simulink model "verify_Storage_Type_1_CONF_mdl"  (R2016b)
settings: Solver=ode45  StartTime=0  StopTime=24*3600  MaxStep=600  RelTol=1e-3  EnableMultiTasking=on
undefined symbols (not defined in the file or in its folder): path_carnot
libraries: carnot x7, simulink x2
settings Model: Creator=drhf  LastModifiedBy=drhf
settings DataIOCC: SaveFormat=Array  SignalLoggingSaveFormat=ModelDataLogs
settings OptimizationCC: ExpressionDepthLimit=2147483647  LifeSpan=inf
settings DebuggingCC: UnderspecifiedInitializationDetection=Classic  MergeDetectMultiDrivingBlocksExec=none  SolverPrmCheckMsg=warning  FcnCallInpInsideContextMsg=warning  StateNameClashWarn=warning  SFUnexpectedBacktrackingDiag=warning  SFNoUnconditionalDefaultTransitionDiag=warning  SFExecutionAtInitializationDiag=none
settings HardwareCC: ProdBitPerPointer=32  ProdBitPerSizeT=32  ProdBitPerPtrDiffT=32  ProdLargestAtomicFloat=None  ProdIntDivRoundTo=Undefined  ProdEndianess=Unspecified  ProdWordSize=32  ProdHWDeviceType=32-bit Generic
settings ModelReferenceCC: PropagateSignalLabelsOutOfModel=off
settings GRTTargetCC: TargetLangStandard=C89/C90 (ANSI)  GeneratePreprocessorConditionals=Disable all  CombineOutputUpdateFcns=off  GRTInterface=on
settings ConfigComp: CovMetricSettings=dw  CovHtmlReporting=on  CovSaveCumulativeToWorkspaceVar=on  CovSaveSingleToWorkspaceVar=on  CovExternalEMLEnable=off

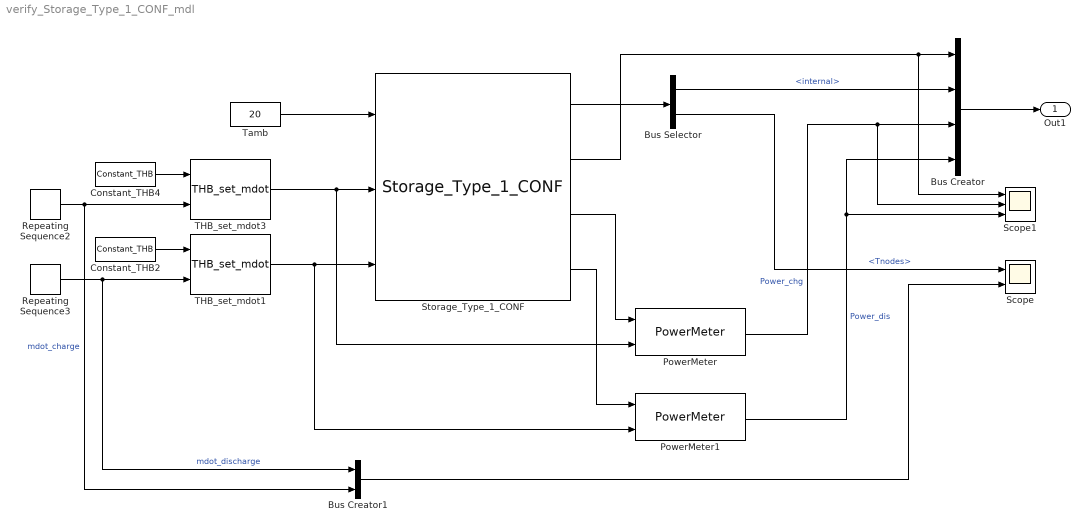
== system verify_Storage_Type_1_CONF_mdl ==
  Bus Creator : BusCreator  Inputs=4
  Bus Creator1 : BusCreator  Inputs=2
  Bus Selector : BusSelector  OutputSignals=energy.internal,Tnodes
  Constant_THB2 : carnot/Source/Simple/Constant_THB  t=10  mdot=100/3600  p=1e5  mID=Full Pressure Drop with Static Height  fluid=Water  mix=0  mix2=0  mix3=0  dia=0.02  hgt=0
  Constant_THB4 : carnot/Source/Simple/Constant_THB  t=55  mdot=0*100/3600  p=1e5  mID=Full Pressure Drop with Static Height  fluid=Water  mix=0  mix2=0  mix3=0  dia=0.02  hgt=0
  PowerMeter : carnot/Control/PowerMeter
  PowerMeter1 : carnot/Control/PowerMeter
  Repeating Sequence2 : simulink/Sources/Repeating Sequence  rep_seq_t=[ 0 3600 3600+eps(3600) 7200 7200+eps(7200) 10440 10440+eps(10440) 11160]  rep_seq_y=[ 0.12 0.12 0.15+0*eps(3600) 0.15 0.1+0*eps(7200) 0.1 0+0*eps(10440) 0]
  Repeating Sequence3 : simulink/Sources/Repeating Sequence  rep_seq_t=[ 0 3600 3600+eps(3600) 7200 7200+eps(7200) 10800]  rep_seq_y=[ 0.12 0.12 0.1+0*eps(3600) 0.1 0.15+0*eps(7200) 0.15]
  Scope : Scope  NumInputPorts=2
  Scope1 : Scope  NumInputPorts=3
  Storage_Type_1_CONF : carnot/Storage/Thermal/Storage_Type_1_CONF  t0=[10:5:55]  hgt=1.5279  stgtype=1  tini=[10 15 20 25 30 35 40 45 50 55]  mpts=[1 2 3 4 5 6 7 8 9 10]  PathName=fullfile(path_carnot('libsl'),'Storage','Thermal','Storage_Type_1_CONF','parameter_set')  FileName='StorageType1_300_L.mat'  userPath=off  userParam=off  uwall=1  ubot=1  utop=1  axcond=1  volume=0.3  dia=0.5  standing=standing cylinder  nodes=10  mpoints=10  Tsensor=0.5  pipe1inlet=1  pipe1outlet=0  pipe1dia=0.03  pipe2inlet=0  pipe2outlet=1  pipe2dia=0.03
  THB_set_mdot1 : carnot/Source/Simple/THB_set_mdot
  THB_set_mdot3 : carnot/Source/Simple/THB_set_mdot
  Tamb : Constant  Value=20
  Out1 : Outport
  wires:
  Bus Creator/1 -> Out1/1
  Tamb/1 -> Storage_Type_1_CONF/1
  THB_set_mdot1/1 -> Storage_Type_1_CONF/3, PowerMeter1/2
  Constant_THB2/1 -> THB_set_mdot1/1
  Storage_Type_1_CONF/4 -> PowerMeter1/1
  PowerMeter/1 -> Scope1/2, Bus Creator/3  "Power_chg"
  PowerMeter1/1 -> Bus Creator/4, Scope1/3  "Power_dis"
  Storage_Type_1_CONF/2 -> Scope1/1, Bus Creator/1
  Bus Selector/1 -> Bus Creator/2  "<internal>"
  Constant_THB4/1 -> THB_set_mdot3/1
  Repeating Sequence2/1 -> Bus Creator1/2, THB_set_mdot3/2  "mdot_charge"
  THB_set_mdot3/1 -> Storage_Type_1_CONF/2, PowerMeter/2
  Storage_Type_1_CONF/1 -> Bus Selector/1
  Storage_Type_1_CONF/3 -> PowerMeter/1
  Bus Selector/2 -> Scope/1  "<Tnodes>"
  Repeating Sequence3/1 -> Bus Creator1/1, THB_set_mdot1/2  "mdot_discharge"
  Bus Creator1/1 -> Scope/2
